simulink model "model"  (R2020a)
settings: Solver=VariableStepAuto  StartTime=0.0  StopTime=10.0  RelTol=1e-3
settings Model: Creator=Avengers  LastModifiedBy=Avengers

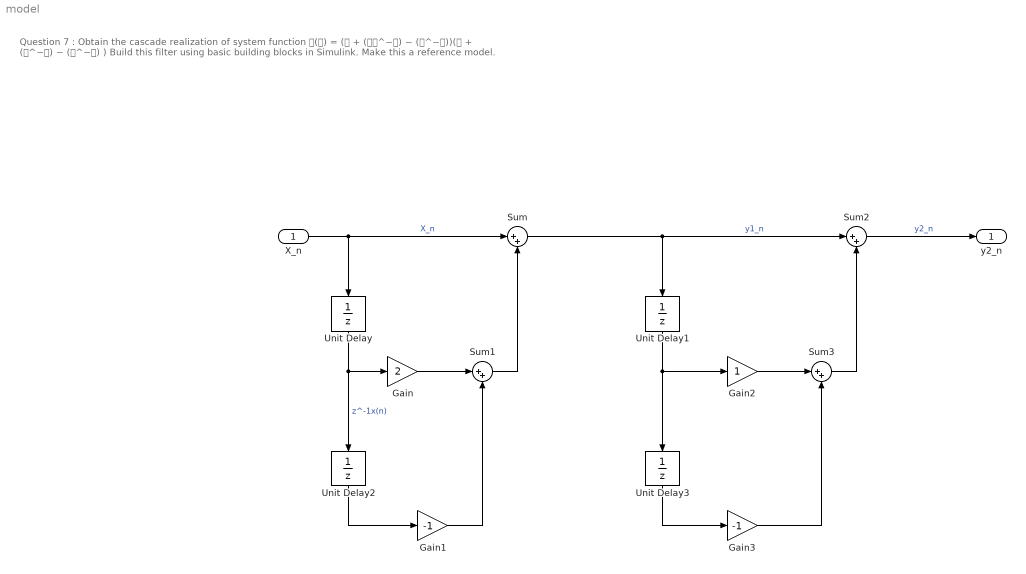
== system model ==
  note: Question 7 :
      | Obtain the cascade realization of system function
      | 𝐇(𝐳) = (𝟏 + (𝟐𝐳^−𝟏) − (𝐳^−𝟐))(𝟏 + (𝐳^−𝟏) − (𝐳^−𝟐) )
      | Build this filter using basic building blocks in Simulink. Make this a reference model.
  X_n : Inport  OutDataTypeStr=double  PortDimensions=1  SampleTime=[0.20000000000000001,0]
  Gain : Gain  Gain=2
  Gain1 : Gain  Gain=-1
  Gain2 : Gain
  Gain3 : Gain  Gain=-1
  Sum{,1..3} (4 alike) : Sum  Inputs=|++
  Unit Delay{,1..3} (4 alike) : UnitDelay  SampleTime=-1  HasFrameUpgradeWarning=on
  y2_n : Outport  OutDataTypeStr=double  PortDimensions=1  SampleTime=[0.20000000000000001,0]
  wires:
  X_n/1 -> Sum/1, Unit Delay/1  "X_n"
  Gain1/1 -> Sum1/2
  Gain3/1 -> Sum3/2
  Unit Delay2/1 -> Gain1/1
  Unit Delay1/1 -> Unit Delay3/1, Gain2/1
  Unit Delay/1 -> Unit Delay2/1, Gain/1  "z^-1x(n)"
  Unit Delay3/1 -> Gain3/1
  Sum3/1 -> Sum2/2
  Gain/1 -> Sum1/1
  Sum1/1 -> Sum/2
  Gain2/1 -> Sum3/1
  Sum/1 -> Unit Delay1/1, Sum2/1  "y1_n"
  Sum2/1 -> y2_n/1  "y2_n"
